simulink model "ROMICL"  (R2022b)
settings: Solver=VariableStepAuto  StartTime=0.0  StopTime=10.0  RelTol=1e-3
undefined symbols (not defined in the file): deltaT, k, k_a, k_d, k_ff, k_i, k_m, k_p, tau_m
settings Model: Creator=ritvi  LastModifiedBy=ritvi

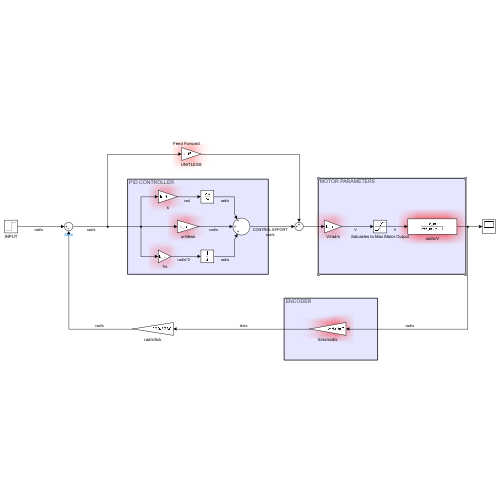
[thumbnail: Simulink's stored preview of the top-level diagram]
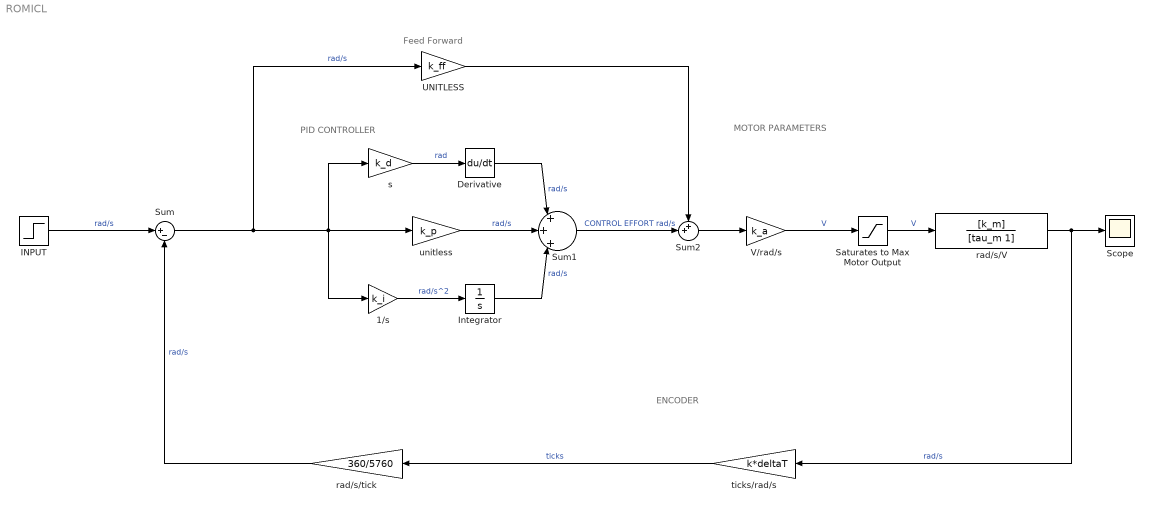
== system ROMICL ==
  note: ENCODER
  note: MOTOR PARAMETERS
  note: Feed Forward
  note: PID CONTROLLER
  1/s : Gain  Gain=k_i
  Derivative : Derivative
  INPUT : Step  SampleTime=0
  Integrator : Integrator
  Saturates to Max Motor Output : Saturate
  Scope : Scope
  Sum : Sum  Inputs=|+-
  Sum1 : Sum  Inputs=|+|+|+|
  Sum2 : Sum  Inputs=++|
  UNITLESS : Gain  Gain=k_ff
  V/rad/s : Gain  Gain=k_a
  rad/s/V : TransferFcn  Numerator=[k_m]  Denominator=[tau_m 1]
  rad/s/tick : Gain  Gain=360/5760
  s : Gain  Gain=k_d
  ticks/rad/s : Gain  Gain=k*deltaT
  unitless : Gain  Gain=k_p
  wires:
  Sum/1 -> UNITLESS/1, s/1, 1/s/1, unitless/1  "rad/s"
  s/1 -> Derivative/1  "rad"
  1/s/1 -> Integrator/1  "rad/s^2"
  Integrator/1 -> Sum1/3  "rad/s"
  unitless/1 -> Sum1/2  "rad/s"
  Derivative/1 -> Sum1/1  "rad/s"
  Sum1/1 -> Sum2/2  "CONTROL EFFORT rad/s"
  UNITLESS/1 -> Sum2/1
  Sum2/1 -> V/rad/s/1
  V/rad/s/1 -> Saturates to Max Motor Output/1  "V"
  Saturates to Max Motor Output/1 -> rad/s/V/1  "V"
  INPUT/1 -> Sum/1  "rad/s"
  rad/s/V/1 -> Scope/1, ticks/rad/s/1  "rad/s"
  ticks/rad/s/1 -> rad/s/tick/1  "ticks"
  rad/s/tick/1 -> Sum/2  "rad/s"
